simulink model "model"  (R2020b)
settings: Solver=VariableStepAuto  StartTime=0.0  StopTime=10.0  RelTol=1e-3
values from neighbouring files (symbols this model uses):
  state0 = [1;0;0]    [runme.m]
settings Model: Creator=fulvioforni  LastModifiedBy=fulvioforni

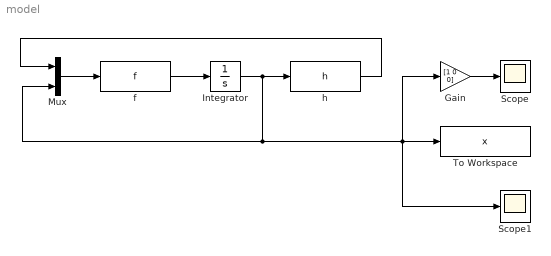
== system model ==
  Gain : Gain  Gain=[1 0 0]
  Integrator : Integrator  InitialCondition=state0
  Mux : Mux  Inputs=2
  Scope : Scope
  Scope1 : Scope
  To Workspace : ToWorkspace  VariableName=x  SaveFormat=Timeseries  SampleTime=-1
  f : MATLABFcn  MATLABFcn=f
  h : MATLABFcn  MATLABFcn=h
  wires:
  f/1 -> Integrator/1
  Integrator/1 -> Scope1/1, Gain/1, To Workspace/1, Mux/2, h/1
  Mux/1 -> f/1
  Gain/1 -> Scope/1
  h/1 -> Mux/1
